simulink model "lab3"  (R2023a)
settings: Solver=VariableStepAuto  StartTime=0.0  StopTime=0.04  RelTol=1e-3
libraries: spsACVoltageSourceLib x3, spsCurrentMeasurementLib x3, spsRMSLib x3, spsGroundLib x2, eePowerMeasurement x2, spsVoltageMeasurementLib x2, spsThreePhaseSeriesRLCBranchLib x1, spsThreePhaseVIMeasurementLib x1, sps_lib x1
settings Model: Creator=HP  LastModifiedBy=HP

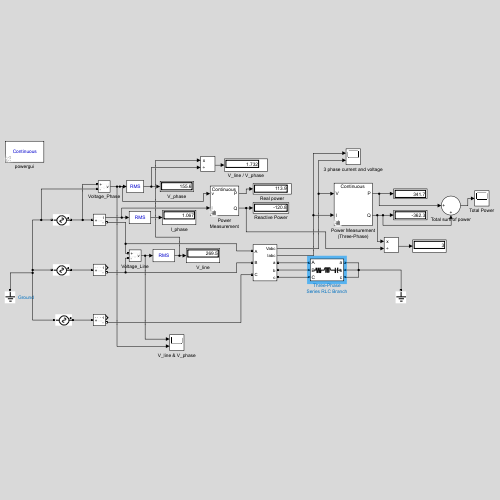
[thumbnail: Simulink's stored preview of the top-level diagram]
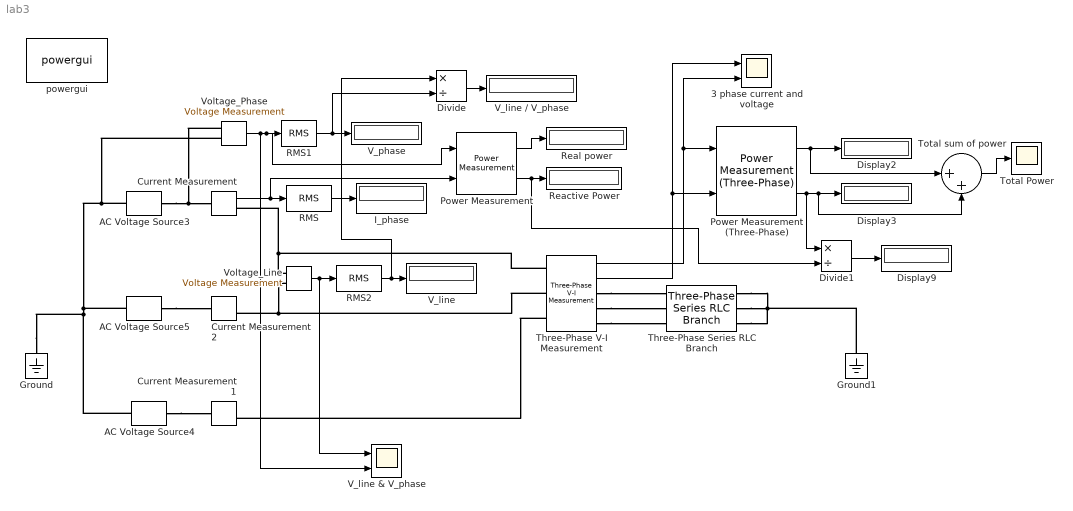
== system lab3 ==
  3 phase current and voltage : Scope  NumInputPorts=2
  AC Voltage Source3 : spsACVoltageSourceLib/AC Voltage Source  Amplitude=220  Phase=0  Frequency=50  SampleTime=0  Measurements=None  BusType=swing  Pref=10e3  Qref=0  Qmin=-inf  Qmax=+inf
  AC Voltage Source4 : spsACVoltageSourceLib/AC Voltage Source  Amplitude=220  Phase=-240  Frequency=50  SampleTime=0  Measurements=None  BusType=swing  Pref=10e3  Qref=0  Qmin=-inf  Qmax=+inf
  AC Voltage Source5 : spsACVoltageSourceLib/AC Voltage Source  Amplitude=220  Phase=-120  Frequency=50  SampleTime=0  Measurements=None  BusType=swing  Pref=10e3  Qref=0  Qmin=-inf  Qmax=+inf
  Current Measurement : spsCurrentMeasurementLib/Current Measurement  PhasorSimulation=off  OutputType=Complex  PSBequivalent=0
  Current Measurement1 : spsCurrentMeasurementLib/Current Measurement  PhasorSimulation=off  OutputType=Complex  PSBequivalent=0
  Current Measurement2 : spsCurrentMeasurementLib/Current Measurement  PhasorSimulation=off  OutputType=Complex  PSBequivalent=0
  Display2 : Display
      settings: Decimation=5
  Display3 : Display
  Display9 : Display
  Divide : Product  Inputs=*/
  Divide1 : Product  Inputs=*/
  Ground : spsGroundLib/Ground  LConnTagsString=a
  Ground1 : spsGroundLib/Ground  LConnTagsString=a
  I_phase : Display
  Power Measurement : eePowerMeasurement/Power Measurement  LabelModeActiveChoice=Continuous  F=50  K=[1]  Ts=0
  Power Measurement (Three-Phase) : eePowerMeasurement/Power Measurement (Three-Phase)  LabelModeActiveChoice=Continuous  F=50  K=[1]  Seq=Positive  Ts=0
  RMS : spsRMSLib/RMS  TrueRMS=on  Freq=50  RMSInit=120  Ts=0
  RMS1 : spsRMSLib/RMS  TrueRMS=on  Freq=50  RMSInit=120  Ts=0
  RMS2 : spsRMSLib/RMS  TrueRMS=on  Freq=50  RMSInit=120  Ts=0
  Reactive Power : Display
  Real power : Display
  Three-Phase Series RLC Branch : spsThreePhaseSeriesRLCBranchLib/Three-Phase Series RLC Branch  LConnTagsString=A|B|C  RConnTagsString=A|B|C  BranchType=RLC  Resistance=100  Inductance=2e-4  Capacitance=3e-5  Measurements=None
  Three-Phase V-I Measurement : spsThreePhaseVIMeasurementLib/Three-Phase V-I Measurement  VoltageMeasurement=phase-to-ground  SetLabelV=off  LabelV=Vabc  Vpu=off  VpuLL=off  CurrentMeasurement=yes  SetLabelI=off  LabelI=Iabc  Ipu=off  Pbase=100e6  Vbase=500e3  OutputType=Complex  PhasorSimulation=off  PSBequivalent=0
  Total Power : Scope
  Total sum of power : Sum  Inputs=|++
  V_line : Display
  V_line & V_phase : Scope  NumInputPorts=2
  V_line / V_phase : Display
  V_phase : Display
  Voltage_Line : spsVoltageMeasurementLib/Voltage Measurement  PhasorSimulation=off  OutputType=Complex  PSBequivalent=0
  Voltage_Phase : spsVoltageMeasurementLib/Voltage Measurement  PhasorSimulation=off  OutputType=Complex  PSBequivalent=0
  powergui : sps_lib/powergui  Priority=1  SimulationMode=Continuous  SampleTime=50e-6  frequency=60  Iterations=50  frequencyindice=50  Pbase=100e6  ErrMax=1e-4  UnitsV=kV  UnitsW=MW  buscounter=0  FunctionMessages=off  echomessages=off  EnableUseOfTLC=off  CurrentSourceSwitches=off  DisableSnubberDevices=off  DisableRonSwitches=off  DisableVfSwitches=off  DisplayEquations=off  AutomaticDiscreteSolvers=off  SolverType=Tustin/Backward Euler (TBE)  Interpol=off  ExternalGateDelay=off  methode=off  Ts=100  x0status=blocks  SPID=on  SwTol=0  HookPort=off  NonlinearTolerance=1e-4  nMaxIteration=100  ContinueOnMaxIteration=off  RestoreLinks=warning  ResistiveCurrentMeasurement=off  Frange=[0:2:500]  Ylog=off  Xlog=on  ShowGrid=off  save=off  variable=ZData  structure=0  ZoomFFT=off  StartTime=0.0  cycles=1  DisplayStyle=1  fundamental=60  FreqAxis=off  MaxFrequency=1000  frequencyindicesteady=1  RmsSteady=1  display=off
  wires:
  Three-Phase V-I Measurement/1 -> 3 phase current and voltage/2, Power Measurement (Three-Phase)/1
  Three-Phase V-I Measurement/2 -> 3 phase current and voltage/1, Power Measurement (Three-Phase)/2
  Current Measurement/1 -> Power Measurement/2, RMS/1
  RMS/1 -> I_phase/1
  Voltage_Phase/1 -> V_line & V_phase/2, Power Measurement/1, RMS1/1
  RMS1/1 -> Divide/2, V_phase/1
  Power Measurement (Three-Phase)/1 -> Total sum of power/1, Display2/1
  Power Measurement (Three-Phase)/2 -> Divide1/1, Display3/1, Total sum of power/2
  RMS2/1 -> Divide/1, V_line/1
  Voltage_Line/1 -> V_line & V_phase/1, RMS2/1
  Power Measurement/1 -> Real power/1
  Divide1/1 -> Display9/1
  Power Measurement/2 -> Divide1/2, Reactive Power/1
  Total sum of power/1 -> Total Power/1
  Divide/1 -> V_line / V_phase/1
  connections:
  Ground/LConn1 -- Voltage_Phase/LConn2 -- AC Voltage Source3/LConn1 -- AC Voltage Source5/LConn1 -- AC Voltage Source4/LConn1
  AC Voltage Source3/RConn1 -- Current Measurement/LConn1 -- Voltage_Phase/LConn1
  Three-Phase V-I Measurement/LConn1 -- Voltage_Line/LConn1 -- Current Measurement/RConn1
  Three-Phase V-I Measurement/LConn2 -- Voltage_Line/LConn2 -- Current Measurement2/RConn1
  AC Voltage Source5/RConn1 -- Current Measurement2/LConn1
  AC Voltage Source4/RConn1 -- Current Measurement1/LConn1
  Three-Phase V-I Measurement/LConn3 -- Current Measurement1/RConn1
  Three-Phase Series RLC Branch/RConn1 -- Ground1/LConn1 -- Three-Phase Series RLC Branch/RConn3 -- Three-Phase Series RLC Branch/RConn2
  Three-Phase V-I Measurement/RConn1 -- Three-Phase Series RLC Branch/LConn1
  Three-Phase V-I Measurement/RConn2 -- Three-Phase Series RLC Branch/LConn2
  Three-Phase V-I Measurement/RConn3 -- Three-Phase Series RLC Branch/LConn3
